simulink model "CubeSatT"  (R2024b)
settings: Solver=ode8  StartTime=0.0  StopTime=10000.0  FixedStep=0.01  RelTol=1e-3
undefined symbols (not defined in the file or in its folder): act, env, flag, IC, orb, sat, sens
libraries: matrix_library x15, simulink_extras x5
(part 2 of 3)

== system CubeSatT/Real World/DKE (Dynamics Kinematics Environment)/Kinematics/Kepler Integrator1 ==
  Add : Sum  Inputs=+-
  Add1 : Sum
  Add2 : Sum
  Clock : Clock
  Constant : Constant  Value=IC.theta
  Constant1 : Constant  Value=3/2
  Constant2 : Constant
  Constant3 : Constant  Value=2
  Constant4 : Constant  Value=orb.e
  Constant5 : Constant  Value=2
  Constant6 : Constant
  Constant7 : Constant  Value=IC.OM
  Constant8 : Constant  Value=2*pi
  Cosh : Trigonometry  Operator=cos
  Divide : Product  Inputs=*/
  Gain : Gain  Gain=orb.n
  Gain1 : Gain  Gain=orb.e
  Gain2 : Gain  Gain=orb.OMprec
  Integrator : Integrator  InitialConditionSource=external  WrapState=on  WrappedStateUpperValue=2*pi  WrappedStateLowerValue=0
  Mod : Math  Operator=mod
  Power : Math  Operator=pow
  Power1 : Math  Operator=pow
  Power2 : Math  Operator=pow
  th : Outport
  OM : Outport  Port=2
  wires:
  Constant/1 -> Integrator/2
  Integrator/1 -> Cosh/1, th/1
  Divide/1 -> Integrator/1
  Power/1 -> Divide/2
  Constant1/1 -> Power/2
  Constant2/1 -> Add/1
  Add/1 -> Power/1
  Power1/1 -> Add/2
  Constant3/1 -> Power1/2
  Constant4/1 -> Power1/1
  Gain/1 -> Divide/1
  Power2/1 -> Gain/1
  Constant5/1 -> Power2/2
  Add1/1 -> Power2/1
  Constant6/1 -> Add1/1
  Gain1/1 -> Add1/2
  Cosh/1 -> Gain1/1
  Constant7/1 -> Add2/2
  Gain2/1 -> Add2/1
  Clock/1 -> Gain2/1
  Add2/1 -> Mod/1
  Constant8/1 -> Mod/2
  Mod/1 -> OM/1

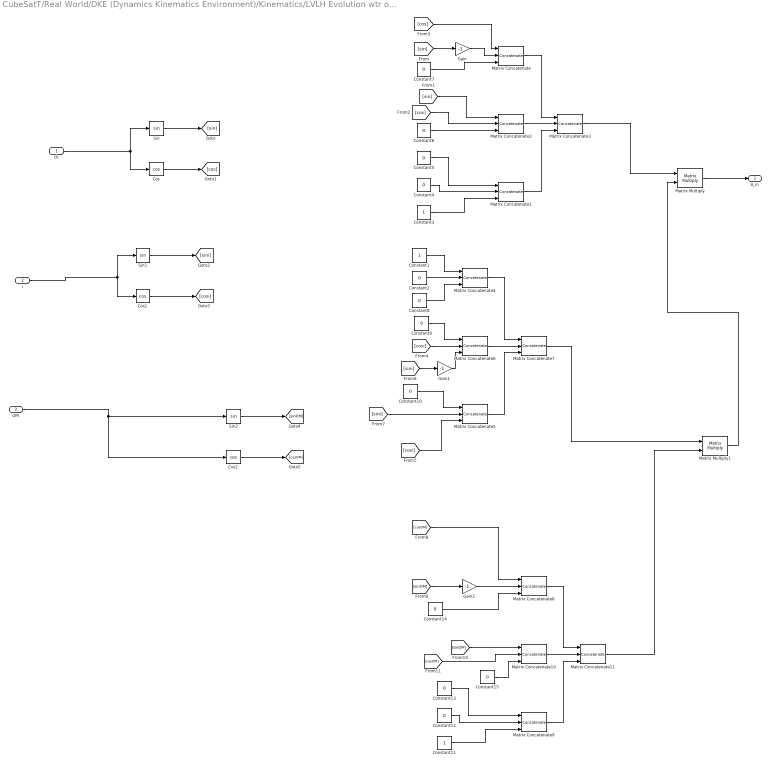
== system CubeSatT/Real World/DKE (Dynamics Kinematics Environment)/Kinematics/LVLH Evolution wtr of Earth ==
  th : Inport
  i : Inport  Port=2
  OM : Inport  Port=3
  Constant1 : Constant
  Constant{2,4..10,12..15} (12 alike) : Constant  Value=0
  Constant11 : Constant
  Constant3 : Constant
  Cos : Trigonometry  Operator=cos
  Cos1 : Trigonometry  Operator=cos
  Cos2 : Trigonometry  Operator=cos
  Gain : Gain  Gain=-1
  Gain1 : Gain  Gain=-1
  Gain2 : Gain  Gain=-1
  Matrix Concatenate{,1..2,4..6,8..10} (9 alike) : Concatenate  NumInputs=3  Mode=Multidimensional array
  Matrix Concatenate11 : Concatenate  NumInputs=3  Mode=Multidimensional array  ConcatenateDimension=2
  Matrix Concatenate3 : Concatenate  NumInputs=3  Mode=Multidimensional array  ConcatenateDimension=2
  Matrix Concatenate7 : Concatenate  NumInputs=3  Mode=Multidimensional array  ConcatenateDimension=2
  Matrix Multiply : Product  Multiplication=Matrix(*)
  Matrix Multiply1 : Product  Multiplication=Matrix(*)
  Sin : Trigonometry
  Sin1 : Trigonometry
  Sin2 : Trigonometry
  A_ln : Outport
  wires:
  Cos/1 -> [cos]
  Matrix Concatenate1/1 -> Matrix Concatenate3/3
  th/1 -> Cos/1, Sin/1
  Matrix Concatenate/1 -> Matrix Concatenate3/1
  Constant5/1 -> Matrix Concatenate1/1
  Constant3/1 -> Matrix Concatenate1/3
  [cos] -> Matrix Concatenate/1
  Sin/1 -> [sin]
  Constant6/1 -> Matrix Concatenate2/3
  Constant7/1 -> Matrix Concatenate/3
  Constant4/1 -> Matrix Concatenate1/2
  Matrix Concatenate2/1 -> Matrix Concatenate3/2
  [cos] -> Matrix Concatenate2/2
  [sin] -> Matrix Concatenate2/1
  Gain/1 -> Matrix Concatenate/2
  [sin] -> Gain/1
  Cos1/1 -> [cosi]
  Sin1/1 -> [sini]
  i/1 -> Cos1/1, Sin1/1
  Matrix Multiply/1 -> A_ln/1
  Matrix Concatenate3/1 -> Matrix Multiply/1
  Matrix Concatenate6/1 -> Matrix Concatenate7/2
  Matrix Concatenate5/1 -> Matrix Concatenate7/3
  Matrix Concatenate4/1 -> Matrix Concatenate7/1
  Constant1/1 -> Matrix Concatenate4/1
  Constant2/1 -> Matrix Concatenate4/2
  Constant8/1 -> Matrix Concatenate4/3
  Constant9/1 -> Matrix Concatenate6/1
  Constant10/1 -> Matrix Concatenate5/1
  [cosi] -> Matrix Concatenate5/3
  [cosi] -> Matrix Concatenate6/2
  [sini] -> Matrix Concatenate5/2
  [sini] -> Gain1/1
  Gain1/1 -> Matrix Concatenate6/3
  Matrix Multiply1/1 -> Matrix Multiply/2
  Matrix Concatenate7/1 -> Matrix Multiply1/1
  OM/1 -> Cos2/1, Sin2/1
  Cos2/1 -> [cosOM]
  Sin2/1 -> [sinOM]
  Matrix Concatenate10/1 -> Matrix Concatenate11/2
  Matrix Concatenate9/1 -> Matrix Concatenate11/3
  Matrix Concatenate8/1 -> Matrix Concatenate11/1
  Matrix Concatenate11/1 -> Matrix Multiply1/2
  Constant13/1 -> Matrix Concatenate9/1
  Constant11/1 -> Matrix Concatenate9/3
  Constant12/1 -> Matrix Concatenate9/2
  Gain2/1 -> Matrix Concatenate8/2
  Constant14/1 -> Matrix Concatenate8/3
  [cosOM] -> Matrix Concatenate8/1
  [sinOM] -> Gain2/1
  [sinOM] -> Matrix Concatenate10/1
  [cosOM] -> Matrix Concatenate10/2
  Constant15/1 -> Matrix Concatenate10/3

== system CubeSatT/Real World/DKE (Dynamics Kinematics Environment)/Kinematics/SpaceCraft position wrt ECI ==
  th : Inport
  OM : Inport  Port=2
  Add : Sum
  Add1 : Sum  Inputs=+-
  Constant{1,7..10,12..15} (9 alike) : Constant  Value=0
  Constant{2..3,11,16} (4 alike) : Constant
  Constant4 : Constant  Value=2
  Constant5 : Constant  Value=orb.e
  Constant6 : Constant  Value=orb.i
  Cos{1..4} (4 alike) : Trigonometry  Operator=cos
  Divide : Product  Inputs=*/
  Gain : Gain  Gain=orb.e
  Gain1 : Gain  Gain=orb.a
  Gain2 : Gain  Gain=-1
  Gain3 : Gain  Gain=-1
  Matrix Concatenate{,4..6,8..10} (7 alike) : Concatenate  NumInputs=3  Mode=Multidimensional array
  Matrix Concatenate11 : Concatenate  NumInputs=3  Mode=Multidimensional array  ConcatenateDimension=2
  Matrix Concatenate7 : Concatenate  NumInputs=3  Mode=Multidimensional array  ConcatenateDimension=2
  Matrix Multiply : Product  Multiplication=Matrix(*)
  Matrix Multiply1 : Product  Multiplication=Matrix(*)
  Power : Math  Operator=pow
  Product2 : Product
  Sin1 : Trigonometry
  Sin2 : Trigonometry
  Sin3 : Trigonometry
  Transpose : Math  Operator=transpose
  r_n : Outport
  wires:
  Cos1/1 -> Matrix Concatenate/1
  th/1 -> Cos2/1, Sin1/1, Cos1/1
  Sin1/1 -> Matrix Concatenate/2
  Product2/1 -> r_n/1
  Divide/1 -> Product2/2
  Constant2/1 -> Add/1
  Add/1 -> Divide/2
  Cos2/1 -> Gain/1
  Gain/1 -> Add/2
  Constant3/1 -> Add1/1
  Power/1 -> Add1/2
  Constant4/1 -> Power/2
  Constant5/1 -> Power/1
  Add1/1 -> Gain1/1
  Gain1/1 -> Divide/1
  Constant6/1 -> Cos3/1, Sin2/1
  Cos3/1 -> [cosi]
  OM/1 -> Cos4/1, Sin3/1
  Sin2/1 -> [sini]
  Sin3/1 -> [sinOM]
  Cos4/1 -> [cosOM]
  Constant1/1 -> Matrix Concatenate/3
  Matrix Multiply/1 -> Product2/1
  Matrix Concatenate/1 -> Matrix Multiply/2
  Transpose/1 -> Matrix Multiply/1
  Constant15/1 -> Matrix Concatenate10/3
  [sinOM] -> Matrix Concatenate10/1
  [sinOM] -> Gain3/1
  Constant13/1 -> Matrix Concatenate9/1
  Gain2/1 -> Matrix Concatenate6/3
  Matrix Concatenate6/1 -> Matrix Concatenate7/2
  Constant14/1 -> Matrix Concatenate8/3
  [sini] -> Gain2/1
  Constant8/1 -> Matrix Concatenate4/3
  Matrix Concatenate4/1 -> Matrix Concatenate7/1
  [cosi] -> Matrix Concatenate5/3
  Constant9/1 -> Matrix Concatenate6/1
  Constant7/1 -> Matrix Concatenate4/2
  Constant10/1 -> Matrix Concatenate5/1
  Matrix Concatenate8/1 -> Matrix Concatenate11/1
  Matrix Concatenate9/1 -> Matrix Concatenate11/3
  Matrix Concatenate7/1 -> Matrix Multiply1/1
  Constant12/1 -> Matrix Concatenate9/2
  [cosi] -> Matrix Concatenate6/2
  Constant11/1 -> Matrix Concatenate9/3
  Constant16/1 -> Matrix Concatenate4/1
  [cosOM] -> Matrix Concatenate10/2
  Gain3/1 -> Matrix Concatenate8/2
  Matrix Concatenate5/1 -> Matrix Concatenate7/3
  [cosOM] -> Matrix Concatenate8/1
  Matrix Concatenate10/1 -> Matrix Concatenate11/2
  [sini] -> Matrix Concatenate5/2
  Matrix Concatenate11/1 -> Matrix Multiply1/2
  Matrix Multiply1/1 -> Transpose/1

== system CubeSatT/Real World/Hardware Models/Actuators/CMG + Control Logic ==
  Mc_b : Inport
  w_mesured : Inport  Port=2
  w : Inport  Port=3
  A assembler : Subsystem
  Add : Sum
  B assembler : Subsystem
  CMG : Subsystem
  Constant3 : Constant  Value=40
  Cross Product : matrix_library/Cross Product
  Degrees to Radians : simulink_extras/Transformations/Degrees to Radians
  Gain : Gain  Gain=-1
  MATLAB Function : MATLAB Function  TreatAsAtomicUnit=on
  Matrix Multiply : Product  Multiplication=Matrix(*)
  hr : Constant  Value=act.cmg.h  VectorParams1D=off
  Mc : Outport
  wires:
  B assembler/1(B) -> MATLAB Function/1(A)
  Mc_b/1 -> Add/1
  CMG/2(Mc) -> Mc/1
  w_mesured/1 -> Cross Product/1
  w/1 -> CMG/2(w)
  Degrees to Radians/1 -> B assembler/1(beta), A assembler/2(beta)
  CMG/1(delta) -> A assembler/1(delta), B assembler/2(delta)
  Matrix Multiply/1 -> Cross Product/2
  Cross Product/1 -> Add/2
  A assembler/1(A) -> Matrix Multiply/1
  hr/1 -> Matrix Multiply/2
  Add/1 -> MATLAB Function/2(B)
  MATLAB Function/1(y) -> Gain/1
  Constant3/1 -> Degrees to Radians/1
  Gain/1 -> CMG/1(delta_dot)

== system CubeSatT/Real World/Hardware Models/Sensors/MAGNETOMETER ==
  note: Missing errors:
      | -SCALE FACTORS ERROR, we can add it to have a more refined model
  B_b : Inport
  Add : Sum
  Constant : Constant  Value=flag.realsensors
  Constant1 : Constant  Value=sens.mag.A_nonorth
  Constant3 : Constant  Value=sens.mag.A_mis
  Demux1 : Demux  Outputs=3
  Matrix Multiply : Product  Multiplication=Matrix(*)
  MatrixMultiply : Product  Multiplication=Matrix(*)
  Mux1 : Mux  Inputs=3
  Noise x : Subsystem
  Noise y : Subsystem
  Noise z : Subsystem
  Switch : Switch  Criteria=u2 > Threshold  SaturateOnIntegerOverflow=off  InputSameDT=off
  "discretization " : ZeroOrderHold  SampleTime=sens.mag.Ts
  quantization : Quantizer  QuantizationInterval=sens.mag.Quant
  saruration : Saturate  UpperLimit=sens.mag.sat(1,1)  LowerLimit=sens.mag.sat(1,2)
  B_meas_b : Outport
  wires:
  Add/1 -> quantization/1
  saruration/1 -> "discretization "/1
  quantization/1 -> saruration/1
  Constant3/1 -> Matrix Multiply/1
  Matrix Multiply/1 -> MatrixMultiply/2
  Constant1/1 -> MatrixMultiply/1
  MatrixMultiply/1 -> Add/1
  Switch/1 -> B_meas_b/1
  Demux1/3 -> Noise z/1(Bz_real)
  B_b/1 -> Demux1/1, Matrix Multiply/2, [B]
  Demux1/1 -> Noise x/1(Bx_real)
  Noise x/1(Out1) -> Mux1/1
  Noise z/1(Out1) -> Mux1/3
  Noise y/1(Out1) -> Mux1/2
  Mux1/1 -> Add/2
  Demux1/2 -> Noise y/1(By_real)
  [B] -> Switch/3
  Constant/1 -> Switch/2
  "discretization "/1 -> Switch/1

== system CubeSatT/Real World/Hardware Models/Sensors/SS Selector ==
  note: Sensor Switch
  note: Validation and Verification Bus Generator
  note: Take care of selecting which Sun Sensor is
      | seeing the sun at a given moment, prioritising the
      | Fine Sensor on the Top panel
      |
      | TODO :
      | Add a variable to switch weights in Wahba's Problem formulation if Fine Sensor is used
      |
      | Change Log
      | Created 21/12/2024
  Fine SS : Inport
  Course SS 1 : Inport  Port=2
  Course SS 2 : Inport  Port=3
  Course SS 3 : Inport  Port=4
  Course SS 4 : Inport  Port=5
  Bus Creator : BusCreator  Inputs=5
  Norm1 : Subsystem
  Norm2 : Subsystem
  Norm3 : Subsystem
  Norm4 : Subsystem
  Switch{,1..3} (4 alike) : Switch  Criteria=u2 ~= 0  SaturateOnIntegerOverflow=off  InputSameDT=off
  Terminator : Terminator
  S_meas_b : Outport
  vv_SS_bus : Outport  Port=2
  wires:
  Fine SS/1 -> [Fine], Norm1/1(Vector)
  Course SS 1/1 -> [Co1], Norm2/1(Vector)
  Course SS 2/1 -> [Co2], Norm3/1(Vector)
  Course SS 3/1 -> [Co3], Norm4/1(Vector)
  Switch/1 -> S_meas_b/1
  Switch1/1 -> Switch/3
  Norm1/1(Norm) -> [FineN]  "norm_r"
  Norm2/1(Norm) -> [Co1N]  "norm_r"
  Norm3/1(Norm) -> [Co2N]  "norm_r"
  Norm4/1(Norm) -> [Co3N]  "norm_r"
  Course SS 4/1 -> Terminator/1, [Co4]  "norm_r"
  Switch2/1 -> Switch1/3
  Switch3/1 -> Switch2/3
  [Co4] -> Switch3/3
  [Fine] -> Switch/1
  [FineN] -> Switch/2
  [Co1] -> Switch1/1
  [Co1N] -> Switch1/2
  [Co2] -> Switch2/1
  [Co2N] -> Switch2/2
  [Co3] -> Switch3/1
  [Co3N] -> Switch3/2
  Bus Creator/1 -> vv_SS_bus/1
  [Fine] -> Bus Creator/1  "Fine_SS"
  [Co1] -> Bus Creator/2  "Co1_SS"
  [Co2] -> Bus Creator/3  "Co2_SS"
  [Co3] -> Bus Creator/4  "Co3_SS"
  [Co4] -> Bus Creator/5  "Co4_SS"

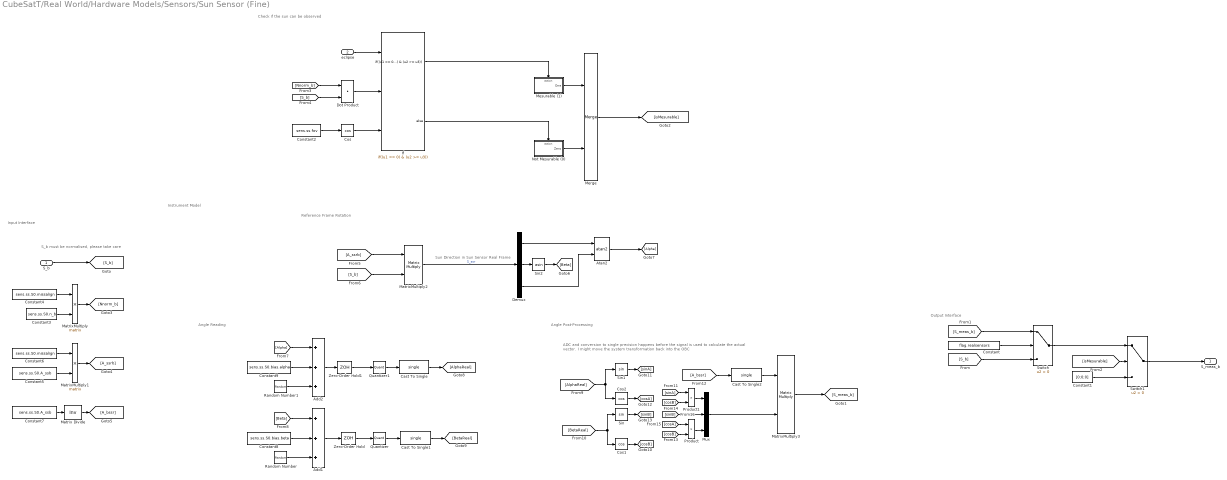
== system CubeSatT/Real World/Hardware Models/Sensors/Sun Sensor (Fine) ==
  note: Instrument Model
  note: Angle Reading
  note: Reference Frame Rotation
  note: ADC and conversion to single precision happens before the signal is used to calculate the actual vector. I might move the system transformation back into the OBC
  note: Sun Direction in Sun Sensor Real Frame
  note: S_b must be normalised, please take care
  note: Input Interface
  note: Output Interface
  note: Check if the sun can be observed
  note: Angle Post-Processing
  S_b : Inport
  eclipse : Inport  Port=2
  Add1 : Sum  Inputs=+++
  Add2 : Sum  Inputs=+++
  Atan2 : Trigonometry  Operator=atan2
  Cast To Single : DataTypeConversion  OutDataTypeStr=single  SaturateOnIntegerOverflow=off  RndMeth=Floor
  Cast To Single1 : DataTypeConversion  OutDataTypeStr=single  SaturateOnIntegerOverflow=off  RndMeth=Floor
  Cast To Single2 : DataTypeConversion  OutDataTypeStr=single  SaturateOnIntegerOverflow=off  RndMeth=Floor
  Constant : Constant  Value=flag.realsensors
  Constant1 : Constant  Value=[0;0;0]
  Constant2 : Constant  Value=sens.ss.fov
  Constant3 : Constant  Value=sens.ss.S0.n_b
  Constant4 : Constant  Value=sens.ss.S0.missalign
  Constant5 : Constant  Value=sens.ss.S0.A_ssb
  Constant6 : Constant  Value=sens.ss.S0.missalign
  Constant7 : Constant  Value=sens.ss.S0.A_ssb
  Constant8 : Constant  Value=sens.ss.S0.bias.beta
  Constant9 : Constant  Value=sens.ss.S0.bias.alpha
  Cos : Trigonometry  Operator=cos
  Cos1 : Trigonometry  Operator=cos
  Cos2 : Trigonometry  Operator=cos
  Demux : Demux  Outputs=3
  Dot Product : DotProduct  OutDataTypeStr=Inherit: Inherit via internal rule
  If : If  NumInputs=3  IfExpression=(u1 == 0) & (u2 >= u3)
  Matrix Divide : Product  Inputs=/  Multiplication=Matrix(*)
  MatrixMultiply{,1..3} (4 alike) : Product  Multiplication=Matrix(*)
  Merge : Merge
  Mesurable (1) : Subsystem  TreatAsAtomicUnit=on
  Mux : Mux  Inputs=3
  Not Mesurable (0) : Subsystem  TreatAsAtomicUnit=on
  Product : Product
  Product1 : Product
  Quantizer : Quantizer  QuantizationInterval=sens.ss.ADC.quanta
  Quantizer1 : Quantizer  QuantizationInterval=sens.ss.ADC.quanta
  Random Number : RandomNumber  Variance=(sens.ss.precision/1.4)^2  Seed=sens.ss.S0.seed.beta  SampleTime=sens.ss.freq
  Random Number1 : RandomNumber  Variance=(sens.ss.precision/1.4)^2  Seed=sens.ss.S0.seed.beta  SampleTime=sens.ss.freq
  Sin : Trigonometry
  Sin1 : Trigonometry
  Sin2 : Trigonometry  Operator=asin
  Switch : Switch  Criteria=u2 > Threshold  SaturateOnIntegerOverflow=off  InputSameDT=off
  Switch1 : Switch  Criteria=u2 > Threshold  SaturateOnIntegerOverflow=off  InputSameDT=off
  Zero-Order Hold : ZeroOrderHold  SampleTime=1/sens.ss.freq
  Zero-Order Hold1 : ZeroOrderHold  SampleTime=1/sens.ss.freq
  S_meas_b : Outport
  wires:
  Constant/1 -> Switch/2
  S_b/1 -> [S_b]
  [S_b] -> Switch/3
  [S_meas_b] -> Switch/1
  eclipse/1 -> If/1
  If/1 -> Mesurable (1)/Action
  If/2 -> Not Mesurable (0)/Action
  Not Mesurable (0)/1(Zero) -> Merge/2
  Mesurable (1)/1(One) -> Merge/1
  Cos/1 -> If/3
  Constant2/1 -> Cos/1
  Dot Product/1 -> If/2
  Merge/1 -> [isMesurable]
  [isMesurable] -> Switch1/2
  [Nnorm_b] -> Dot Product/1
  [S_b] -> Dot Product/2
  Constant4/1 -> MatrixMultiply/1
  MatrixMultiply/1 -> [Nnorm_b]
  Constant3/1 -> MatrixMultiply/2
  Constant1/1 -> Switch1/3
  Switch/1 -> Switch1/1
  Constant6/1 -> MatrixMultiply1/1
  Constant5/1 -> MatrixMultiply1/2
  MatrixMultiply1/1 -> [A_ssrb]
  Constant7/1 -> Matrix Divide/1
  Matrix Divide/1 -> [A_bssr]
  [A_ssrb] -> MatrixMultiply2/1
  [S_b] -> MatrixMultiply2/2
  MatrixMultiply2/1 -> Demux/1  "S_ssr"
  Demux/1 -> Atan2/1
  Demux/3 -> Atan2/2
  Sin2/1 -> [Beta]
  Add2/1 -> Zero-Order Hold1/1
  Add1/1 -> Zero-Order Hold/1
  Quantizer1/1 -> Cast To Single/1
  Zero-Order Hold1/1 -> Quantizer1/1
  Quantizer/1 -> Cast To Single1/1
  Zero-Order Hold/1 -> Quantizer/1
  [Alpha] -> Add2/1
  [Beta] -> Add1/1
  Constant8/1 -> Add1/2
  Constant9/1 -> Add2/2
  Cast To Single/1 -> [AlphaReal]
  Cast To Single1/1 -> [BetaReal]
  Random Number/1 -> Add1/3
  Random Number1/1 -> Add2/3
  Switch1/1 -> S_meas_b/1
  MatrixMultiply3/1 -> [S_meas_b]
  Mux/1 -> MatrixMultiply3/2
  Cast To Single2/1 -> MatrixMultiply3/1
  [A_bssr] -> Cast To Single2/1
  [BetaReal] -> Cos1/1, Sin/1
  Atan2/1 -> [Alpha]
  [AlphaReal] -> Cos2/1, Sin1/1
  Product/1 -> Mux/3
  Product1/1 -> Mux/1
  Demux/2 -> Sin2/1
  Sin1/1 -> [sinA]
  Cos2/1 -> [cosA]
  [sinA] -> Product1/1
  Cos1/1 -> [cosB]
  [cosB] -> Product/2
  [cosB] -> Product1/2
  [cosA] -> Product/1
  Sin/1 -> [sinB]
  [sinB] -> Mux/2

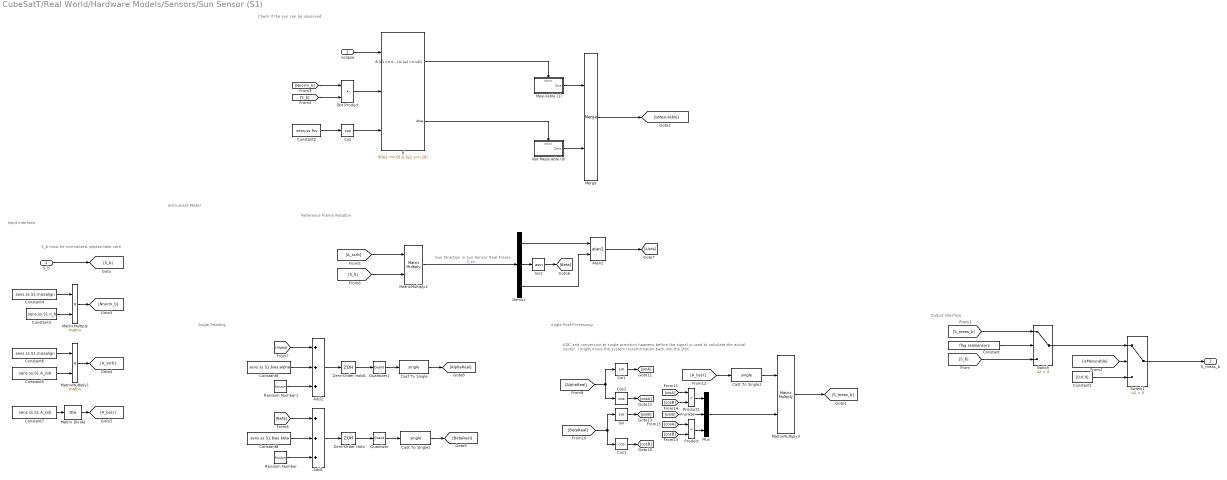
== system CubeSatT/Real World/Hardware Models/Sensors/Sun Sensor (S1) ==
  note: Instrument Model
  note: Angle Reading
  note: Reference Frame Rotation
  note: ADC and conversion to single precision happens before the signal is used to calculate the actual vector. I might move the system transformation back into the OBC
  note: Sun Direction in Sun Sensor Real Frame
  note: S_b must be normalised, please take care
  note: Input Interface
  note: Output Interface
  note: Check if the sun can be observed
  note: Angle Post-Processing
  S_b : Inport
  eclipse : Inport  Port=2
  Add1 : Sum  Inputs=+++
  Add2 : Sum  Inputs=+++
  Atan2 : Trigonometry  Operator=atan2
  Cast To Single : DataTypeConversion  OutDataTypeStr=single  SaturateOnIntegerOverflow=off  RndMeth=Floor
  Cast To Single1 : DataTypeConversion  OutDataTypeStr=single  SaturateOnIntegerOverflow=off  RndMeth=Floor
  Cast To Single2 : DataTypeConversion  OutDataTypeStr=single  SaturateOnIntegerOverflow=off  RndMeth=Floor
  Constant : Constant  Value=flag.realsensors
  Constant1 : Constant  Value=[0;0;0]
  Constant2 : Constant  Value=sens.ss.fov
  Constant3 : Constant  Value=sens.ss.S1.n_b  VectorParams1D=off
  Constant4 : Constant  Value=sens.ss.S1.missalign
  Constant5 : Constant  Value=sens.ss.S1.A_ssb
  Constant6 : Constant  Value=sens.ss.S1.missalign
  Constant7 : Constant  Value=sens.ss.S1.A_ssb
  Constant8 : Constant  Value=sens.ss.S1.bias.beta
  Constant9 : Constant  Value=sens.ss.S1.bias.alpha
  Cos : Trigonometry  Operator=cos
  Cos1 : Trigonometry  Operator=cos
  Cos2 : Trigonometry  Operator=cos
  Demux : Demux  Outputs=3
  Dot Product : DotProduct  OutDataTypeStr=Inherit: Inherit via internal rule
  If : If  NumInputs=3  IfExpression=(u1 == 0) & (u2 >= u3)
  Matrix Divide : Product  Inputs=/  Multiplication=Matrix(*)
  MatrixMultiply{,1..3} (4 alike) : Product  Multiplication=Matrix(*)
  Merge : Merge
  Mesurable (1) : Subsystem  TreatAsAtomicUnit=on
  Mux : Mux  Inputs=3
  Not Mesurable (0) : Subsystem  TreatAsAtomicUnit=on
  Product : Product
  Product1 : Product
  Quantizer : Quantizer  QuantizationInterval=sens.ss.ADC.quanta
  Quantizer1 : Quantizer  QuantizationInterval=sens.ss.ADC.quanta
  Random Number : RandomNumber  Variance=(sens.ss.precision/1.4)^2  Seed=sens.ss.S0.seed.beta  SampleTime=sens.ss.freq
  Random Number1 : RandomNumber  Variance=(sens.ss.precision/1.4)^2  Seed=sens.ss.S0.seed.beta  SampleTime=sens.ss.freq
  Sin : Trigonometry
  Sin1 : Trigonometry
  Sin2 : Trigonometry  Operator=asin
  Switch : Switch  Criteria=u2 > Threshold  SaturateOnIntegerOverflow=off  InputSameDT=off
  Switch1 : Switch  Criteria=u2 > Threshold  SaturateOnIntegerOverflow=off  InputSameDT=off
  Zero-Order Hold : ZeroOrderHold  SampleTime=1/sens.ss.freq
  Zero-Order Hold1 : ZeroOrderHold  SampleTime=1/sens.ss.freq
  S_meas_b : Outport
  wires:
  Constant/1 -> Switch/2
  S_b/1 -> [S_b]
  [S_b] -> Switch/3
  [S_meas_b] -> Switch/1
  eclipse/1 -> If/1
  If/1 -> Mesurable (1)/Action
  If/2 -> Not Mesurable (0)/Action
  Not Mesurable (0)/1(Zero) -> Merge/2
  Mesurable (1)/1(One) -> Merge/1
  Cos/1 -> If/3
  Constant2/1 -> Cos/1
  Dot Product/1 -> If/2
  Merge/1 -> [isMesurable]
  [isMesurable] -> Switch1/2
  [Nnorm_b] -> Dot Product/1
  [S_b] -> Dot Product/2
  Constant4/1 -> MatrixMultiply/1
  MatrixMultiply/1 -> [Nnorm_b]
  Constant3/1 -> MatrixMultiply/2
  Constant1/1 -> Switch1/3
  Switch/1 -> Switch1/1
  Constant6/1 -> MatrixMultiply1/1
  Constant5/1 -> MatrixMultiply1/2
  MatrixMultiply1/1 -> [A_ssrb]
  Constant7/1 -> Matrix Divide/1
  Matrix Divide/1 -> [A_bssr]
  [A_ssrb] -> MatrixMultiply2/1
  [S_b] -> MatrixMultiply2/2
  MatrixMultiply2/1 -> Demux/1  "S_ssr"
  Demux/1 -> Atan2/1
  Demux/3 -> Atan2/2
  Sin2/1 -> [Beta]
  Add2/1 -> Zero-Order Hold1/1
  Add1/1 -> Zero-Order Hold/1
  Quantizer1/1 -> Cast To Single/1
  Zero-Order Hold1/1 -> Quantizer1/1
  Quantizer/1 -> Cast To Single1/1
  Zero-Order Hold/1 -> Quantizer/1
  [Alpha] -> Add2/1
  [Beta] -> Add1/1
  Constant8/1 -> Add1/2
  Constant9/1 -> Add2/2
  Cast To Single/1 -> [AlphaReal]
  Cast To Single1/1 -> [BetaReal]
  Random Number/1 -> Add1/3
  Random Number1/1 -> Add2/3
  Switch1/1 -> S_meas_b/1
  MatrixMultiply3/1 -> [S_meas_b]
  Mux/1 -> MatrixMultiply3/2
  Cast To Single2/1 -> MatrixMultiply3/1
  [A_bssr] -> Cast To Single2/1
  [BetaReal] -> Cos1/1, Sin/1
  Atan2/1 -> [Alpha]
  [AlphaReal] -> Cos2/1, Sin1/1
  Product/1 -> Mux/3
  Product1/1 -> Mux/1
  Demux/2 -> Sin2/1
  Sin1/1 -> [sinA]
  Cos2/1 -> [cosA]
  [sinA] -> Product1/1
  Cos1/1 -> [cosB]
  [cosB] -> Product/2
  [cosB] -> Product1/2
  [cosA] -> Product/1
  Sin/1 -> [sinB]
  [sinB] -> Mux/2

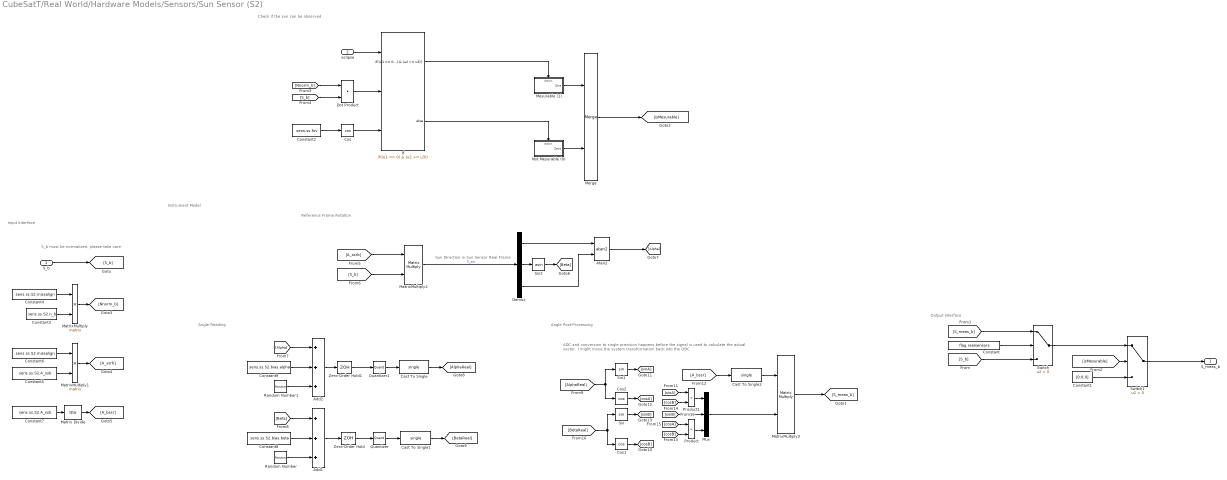
== system CubeSatT/Real World/Hardware Models/Sensors/Sun Sensor (S2) ==
  note: Instrument Model
  note: Angle Reading
  note: Reference Frame Rotation
  note: ADC and conversion to single precision happens before the signal is used to calculate the actual vector. I might move the system transformation back into the OBC
  note: Sun Direction in Sun Sensor Real Frame
  note: S_b must be normalised, please take care
  note: Input Interface
  note: Output Interface
  note: Check if the sun can be observed
  note: Angle Post-Processing
  S_b : Inport
  eclipse : Inport  Port=2
  Add1 : Sum  Inputs=+++
  Add2 : Sum  Inputs=+++
  Atan2 : Trigonometry  Operator=atan2
  Cast To Single : DataTypeConversion  OutDataTypeStr=single  SaturateOnIntegerOverflow=off  RndMeth=Floor
  Cast To Single1 : DataTypeConversion  OutDataTypeStr=single  SaturateOnIntegerOverflow=off  RndMeth=Floor
  Cast To Single2 : DataTypeConversion  OutDataTypeStr=single  SaturateOnIntegerOverflow=off  RndMeth=Floor
  Constant : Constant  Value=flag.realsensors
  Constant1 : Constant  Value=[0;0;0]
  Constant2 : Constant  Value=sens.ss.fov
  Constant3 : Constant  Value=sens.ss.S2.n_b
  Constant4 : Constant  Value=sens.ss.S2.missalign
  Constant5 : Constant  Value=sens.ss.S2.A_ssb
  Constant6 : Constant  Value=sens.ss.S2.missalign  VectorParams1D=off
  Constant7 : Constant  Value=sens.ss.S2.A_ssb
  Constant8 : Constant  Value=sens.ss.S2.bias.beta
  Constant9 : Constant  Value=sens.ss.S2.bias.alpha
  Cos : Trigonometry  Operator=cos
  Cos1 : Trigonometry  Operator=cos
  Cos2 : Trigonometry  Operator=cos
  Demux : Demux  Outputs=3
  Dot Product : DotProduct  OutDataTypeStr=Inherit: Inherit via internal rule
  If : If  NumInputs=3  IfExpression=(u1 == 0) & (u2 >= u3)
  Matrix Divide : Product  Inputs=/  Multiplication=Matrix(*)
  MatrixMultiply{,1..3} (4 alike) : Product  Multiplication=Matrix(*)
  Merge : Merge
  Mesurable (1) : Subsystem  TreatAsAtomicUnit=on
  Mux : Mux  Inputs=3
  Not Mesurable (0) : Subsystem  TreatAsAtomicUnit=on
  Product : Product
  Product1 : Product
  Quantizer : Quantizer  QuantizationInterval=sens.ss.ADC.quanta
  Quantizer1 : Quantizer  QuantizationInterval=sens.ss.ADC.quanta
  Random Number : RandomNumber  Variance=(sens.ss.precision/1.4)^2  Seed=sens.ss.S0.seed.beta  SampleTime=sens.ss.freq
  Random Number1 : RandomNumber  Variance=(sens.ss.precision/1.4)^2  Seed=sens.ss.S0.seed.beta  SampleTime=sens.ss.freq
  Sin : Trigonometry
  Sin1 : Trigonometry
  Sin2 : Trigonometry  Operator=asin
  Switch : Switch  Criteria=u2 > Threshold  SaturateOnIntegerOverflow=off  InputSameDT=off
  Switch1 : Switch  Criteria=u2 > Threshold  SaturateOnIntegerOverflow=off  InputSameDT=off
  Zero-Order Hold : ZeroOrderHold  SampleTime=1/sens.ss.freq
  Zero-Order Hold1 : ZeroOrderHold  SampleTime=1/sens.ss.freq
  S_meas_b : Outport
  wires:
  Constant/1 -> Switch/2
  S_b/1 -> [S_b]
  [S_b] -> Switch/3
  [S_meas_b] -> Switch/1
  eclipse/1 -> If/1
  If/1 -> Mesurable (1)/Action
  If/2 -> Not Mesurable (0)/Action
  Not Mesurable (0)/1(Zero) -> Merge/2
  Mesurable (1)/1(One) -> Merge/1
  Cos/1 -> If/3
  Constant2/1 -> Cos/1
  Dot Product/1 -> If/2
  Merge/1 -> [isMesurable]
  [isMesurable] -> Switch1/2
  [Nnorm_b] -> Dot Product/1
  [S_b] -> Dot Product/2
  Constant4/1 -> MatrixMultiply/1
  MatrixMultiply/1 -> [Nnorm_b]
  Constant3/1 -> MatrixMultiply/2
  Constant1/1 -> Switch1/3
  Switch/1 -> Switch1/1
  Constant6/1 -> MatrixMultiply1/1
  Constant5/1 -> MatrixMultiply1/2
  MatrixMultiply1/1 -> [A_ssrb]
  Constant7/1 -> Matrix Divide/1
  Matrix Divide/1 -> [A_bssr]
  [A_ssrb] -> MatrixMultiply2/1
  [S_b] -> MatrixMultiply2/2
  MatrixMultiply2/1 -> Demux/1  "S_ssr"
  Demux/1 -> Atan2/1
  Demux/3 -> Atan2/2
  Sin2/1 -> [Beta]
  Add2/1 -> Zero-Order Hold1/1
  Add1/1 -> Zero-Order Hold/1
  Quantizer1/1 -> Cast To Single/1
  Zero-Order Hold1/1 -> Quantizer1/1
  Quantizer/1 -> Cast To Single1/1
  Zero-Order Hold/1 -> Quantizer/1
  [Alpha] -> Add2/1
  [Beta] -> Add1/1
  Constant8/1 -> Add1/2
  Constant9/1 -> Add2/2
  Cast To Single/1 -> [AlphaReal]
  Cast To Single1/1 -> [BetaReal]
  Random Number/1 -> Add1/3
  Random Number1/1 -> Add2/3
  Switch1/1 -> S_meas_b/1
  MatrixMultiply3/1 -> [S_meas_b]
  Mux/1 -> MatrixMultiply3/2
  Cast To Single2/1 -> MatrixMultiply3/1
  [A_bssr] -> Cast To Single2/1
  [BetaReal] -> Cos1/1, Sin/1
  Atan2/1 -> [Alpha]
  [AlphaReal] -> Cos2/1, Sin1/1
  Product/1 -> Mux/3
  Product1/1 -> Mux/1
  Demux/2 -> Sin2/1
  Sin1/1 -> [sinA]
  Cos2/1 -> [cosA]
  [sinA] -> Product1/1
  Cos1/1 -> [cosB]
  [cosB] -> Product/2
  [cosB] -> Product1/2
  [cosA] -> Product/1
  Sin/1 -> [sinB]
  [sinB] -> Mux/2

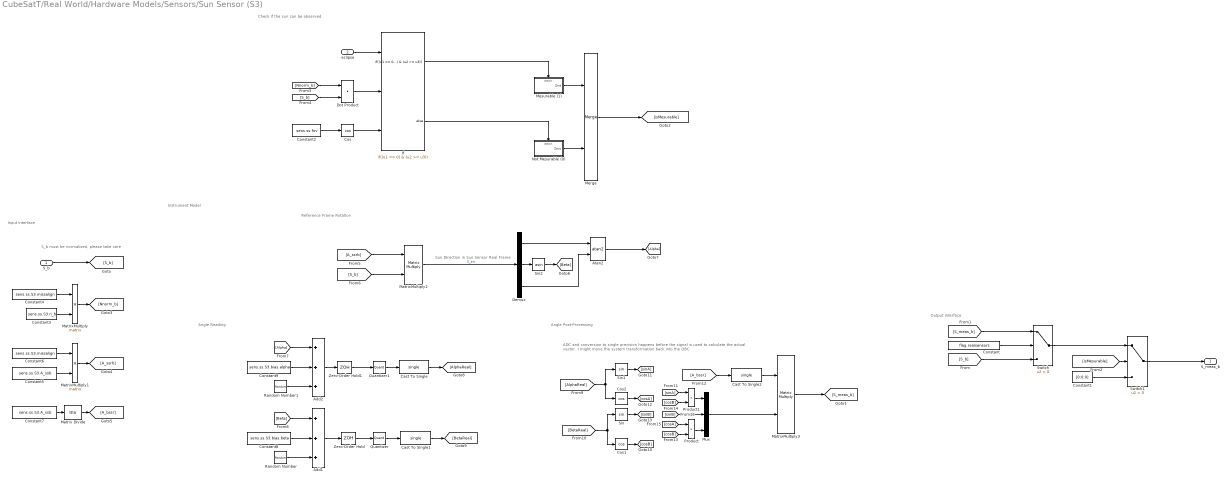
== system CubeSatT/Real World/Hardware Models/Sensors/Sun Sensor (S3) ==
  note: Instrument Model
  note: Angle Reading
  note: Reference Frame Rotation
  note: ADC and conversion to single precision happens before the signal is used to calculate the actual vector. I might move the system transformation back into the OBC
  note: Sun Direction in Sun Sensor Real Frame
  note: S_b must be normalised, please take care
  note: Input Interface
  note: Output Interface
  note: Check if the sun can be observed
  note: Angle Post-Processing
  S_b : Inport
  eclipse : Inport  Port=2
  Add1 : Sum  Inputs=+++
  Add2 : Sum  Inputs=+++
  Atan2 : Trigonometry  Operator=atan2
  Cast To Single : DataTypeConversion  OutDataTypeStr=single  SaturateOnIntegerOverflow=off  RndMeth=Floor
  Cast To Single1 : DataTypeConversion  OutDataTypeStr=single  SaturateOnIntegerOverflow=off  RndMeth=Floor
  Cast To Single2 : DataTypeConversion  OutDataTypeStr=single  SaturateOnIntegerOverflow=off  RndMeth=Floor
  Constant : Constant  Value=flag.realsensors
  Constant1 : Constant  Value=[0;0;0]
  Constant2 : Constant  Value=sens.ss.fov
  Constant3 : Constant  Value=sens.ss.S3.n_b
  Constant4 : Constant  Value=sens.ss.S3.missalign
  Constant5 : Constant  Value=sens.ss.S3.A_ssb
  Constant6 : Constant  Value=sens.ss.S3.missalign
  Constant7 : Constant  Value=sens.ss.S3.A_ssb
  Constant8 : Constant  Value=sens.ss.S3.bias.beta
  Constant9 : Constant  Value=sens.ss.S3.bias.alpha
  Cos : Trigonometry  Operator=cos
  Cos1 : Trigonometry  Operator=cos
  Cos2 : Trigonometry  Operator=cos
  Demux : Demux  Outputs=3
  Dot Product : DotProduct  OutDataTypeStr=Inherit: Inherit via internal rule
  If : If  NumInputs=3  IfExpression=(u1 == 0) & (u2 >= u3)
  Matrix Divide : Product  Inputs=/  Multiplication=Matrix(*)
  MatrixMultiply{,1..3} (4 alike) : Product  Multiplication=Matrix(*)
  Merge : Merge
  Mesurable (1) : Subsystem  TreatAsAtomicUnit=on
  Mux : Mux  Inputs=3
  Not Mesurable (0) : Subsystem  TreatAsAtomicUnit=on
  Product : Product
  Product1 : Product
  Quantizer : Quantizer  QuantizationInterval=sens.ss.ADC.quanta
  Quantizer1 : Quantizer  QuantizationInterval=sens.ss.ADC.quanta
  Random Number : RandomNumber  Variance=(sens.ss.precision/1.4)^2  Seed=sens.ss.S0.seed.beta  SampleTime=sens.ss.freq
  Random Number1 : RandomNumber  Variance=(sens.ss.precision/1.4)^2  Seed=sens.ss.S0.seed.beta  SampleTime=sens.ss.freq
  Sin : Trigonometry
  Sin1 : Trigonometry
  Sin2 : Trigonometry  Operator=asin
  Switch : Switch  Criteria=u2 > Threshold  SaturateOnIntegerOverflow=off  InputSameDT=off
  Switch1 : Switch  Criteria=u2 > Threshold  SaturateOnIntegerOverflow=off  InputSameDT=off
  Zero-Order Hold : ZeroOrderHold  SampleTime=1/sens.ss.freq
  Zero-Order Hold1 : ZeroOrderHold  SampleTime=1/sens.ss.freq
  S_meas_b : Outport
  wires:
  Constant/1 -> Switch/2
  S_b/1 -> [S_b]
  [S_b] -> Switch/3
  [S_meas_b] -> Switch/1
  eclipse/1 -> If/1
  If/1 -> Mesurable (1)/Action
  If/2 -> Not Mesurable (0)/Action
  Not Mesurable (0)/1(Zero) -> Merge/2
  Mesurable (1)/1(One) -> Merge/1
  Cos/1 -> If/3
  Constant2/1 -> Cos/1
  Dot Product/1 -> If/2
  Merge/1 -> [isMesurable]
  [isMesurable] -> Switch1/2
  [Nnorm_b] -> Dot Product/1
  [S_b] -> Dot Product/2
  Constant4/1 -> MatrixMultiply/1
  MatrixMultiply/1 -> [Nnorm_b]
  Constant3/1 -> MatrixMultiply/2
  Constant1/1 -> Switch1/3
  Switch/1 -> Switch1/1
  Constant6/1 -> MatrixMultiply1/1
  Constant5/1 -> MatrixMultiply1/2
  MatrixMultiply1/1 -> [A_ssrb]
  Constant7/1 -> Matrix Divide/1
  Matrix Divide/1 -> [A_bssr]
  [A_ssrb] -> MatrixMultiply2/1
  [S_b] -> MatrixMultiply2/2
  MatrixMultiply2/1 -> Demux/1  "S_ssr"
  Demux/1 -> Atan2/1
  Demux/3 -> Atan2/2
  Sin2/1 -> [Beta]
  Add2/1 -> Zero-Order Hold1/1
  Add1/1 -> Zero-Order Hold/1
  Quantizer1/1 -> Cast To Single/1
  Zero-Order Hold1/1 -> Quantizer1/1
  Quantizer/1 -> Cast To Single1/1
  Zero-Order Hold/1 -> Quantizer/1
  [Alpha] -> Add2/1
  [Beta] -> Add1/1
  Constant8/1 -> Add1/2
  Constant9/1 -> Add2/2
  Cast To Single/1 -> [AlphaReal]
  Cast To Single1/1 -> [BetaReal]
  Random Number/1 -> Add1/3
  Random Number1/1 -> Add2/3
  Switch1/1 -> S_meas_b/1
  MatrixMultiply3/1 -> [S_meas_b]
  Mux/1 -> MatrixMultiply3/2
  Cast To Single2/1 -> MatrixMultiply3/1
  [A_bssr] -> Cast To Single2/1
  [BetaReal] -> Cos1/1, Sin/1
  Atan2/1 -> [Alpha]
  [AlphaReal] -> Cos2/1, Sin1/1
  Product/1 -> Mux/3
  Product1/1 -> Mux/1
  Demux/2 -> Sin2/1
  Sin1/1 -> [sinA]
  Cos2/1 -> [cosA]
  [sinA] -> Product1/1
  Cos1/1 -> [cosB]
  [cosB] -> Product/2
  [cosB] -> Product1/2
  [cosA] -> Product/1
  Sin/1 -> [sinB]
  [sinB] -> Mux/2

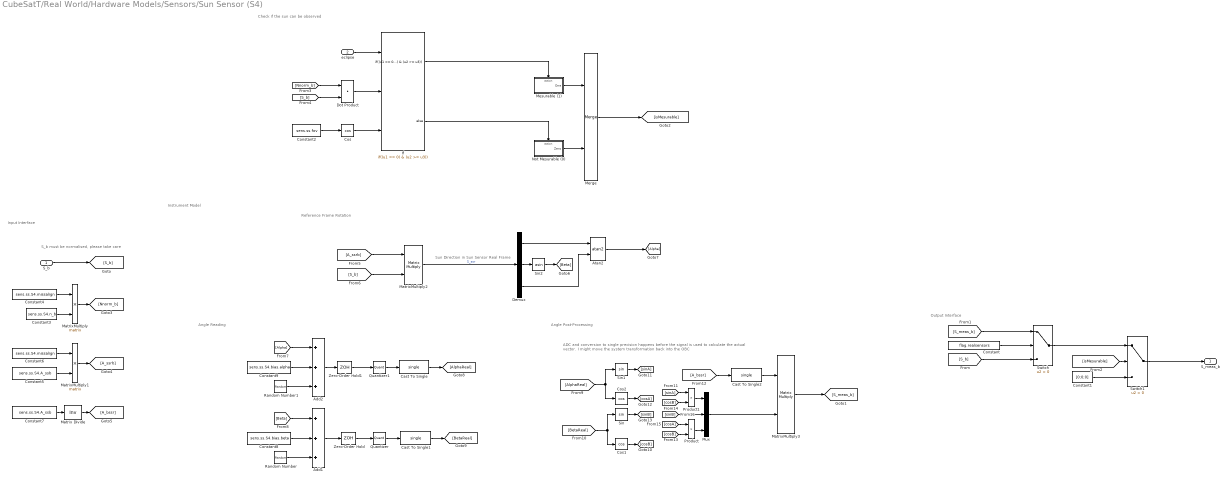
== system CubeSatT/Real World/Hardware Models/Sensors/Sun Sensor (S4) ==
  note: Instrument Model
  note: Angle Reading
  note: Reference Frame Rotation
  note: ADC and conversion to single precision happens before the signal is used to calculate the actual vector. I might move the system transformation back into the OBC
  note: Sun Direction in Sun Sensor Real Frame
  note: S_b must be normalised, please take care
  note: Input Interface
  note: Output Interface
  note: Check if the sun can be observed
  note: Angle Post-Processing
  S_b : Inport
  eclipse : Inport  Port=2
  Add1 : Sum  Inputs=+++
  Add2 : Sum  Inputs=+++
  Atan2 : Trigonometry  Operator=atan2
  Cast To Single : DataTypeConversion  OutDataTypeStr=single  SaturateOnIntegerOverflow=off  RndMeth=Floor
  Cast To Single1 : DataTypeConversion  OutDataTypeStr=single  SaturateOnIntegerOverflow=off  RndMeth=Floor
  Cast To Single2 : DataTypeConversion  OutDataTypeStr=single  SaturateOnIntegerOverflow=off  RndMeth=Floor
  Constant : Constant  Value=flag.realsensors
  Constant1 : Constant  Value=[0;0;0]
  Constant2 : Constant  Value=sens.ss.fov
  Constant3 : Constant  Value=sens.ss.S4.n_b
  Constant4 : Constant  Value=sens.ss.S4.missalign
  Constant5 : Constant  Value=sens.ss.S4.A_ssb
  Constant6 : Constant  Value=sens.ss.S4.missalign
  Constant7 : Constant  Value=sens.ss.S4.A_ssb
  Constant8 : Constant  Value=sens.ss.S4.bias.beta
  Constant9 : Constant  Value=sens.ss.S4.bias.alpha
  Cos : Trigonometry  Operator=cos
  Cos1 : Trigonometry  Operator=cos
  Cos2 : Trigonometry  Operator=cos
  Demux : Demux  Outputs=3
  Dot Product : DotProduct  OutDataTypeStr=Inherit: Inherit via internal rule
  If : If  NumInputs=3  IfExpression=(u1 == 0) & (u2 >= u3)
  Matrix Divide : Product  Inputs=/  Multiplication=Matrix(*)
  MatrixMultiply{,1..3} (4 alike) : Product  Multiplication=Matrix(*)
  Merge : Merge
  Mesurable (1) : Subsystem  TreatAsAtomicUnit=on
  Mux : Mux  Inputs=3
  Not Mesurable (0) : Subsystem  TreatAsAtomicUnit=on
  Product : Product
  Product1 : Product
  Quantizer : Quantizer  QuantizationInterval=sens.ss.ADC.quanta
  Quantizer1 : Quantizer  QuantizationInterval=sens.ss.ADC.quanta
  Random Number : RandomNumber  Variance=(sens.ss.precision/1.4)^2  Seed=sens.ss.S0.seed.beta  SampleTime=sens.ss.freq
  Random Number1 : RandomNumber  Variance=(sens.ss.precision/1.4)^2  Seed=sens.ss.S0.seed.beta  SampleTime=sens.ss.freq
  Sin : Trigonometry
  Sin1 : Trigonometry
  Sin2 : Trigonometry  Operator=asin
  Switch : Switch  Criteria=u2 > Threshold  SaturateOnIntegerOverflow=off  InputSameDT=off
  Switch1 : Switch  Criteria=u2 > Threshold  SaturateOnIntegerOverflow=off  InputSameDT=off
  Zero-Order Hold : ZeroOrderHold  SampleTime=1/sens.ss.freq
  Zero-Order Hold1 : ZeroOrderHold  SampleTime=1/sens.ss.freq
  S_meas_b : Outport
  wires:
  Constant/1 -> Switch/2
  S_b/1 -> [S_b]
  [S_b] -> Switch/3
  [S_meas_b] -> Switch/1
  eclipse/1 -> If/1
  If/1 -> Mesurable (1)/Action
  If/2 -> Not Mesurable (0)/Action
  Not Mesurable (0)/1(Zero) -> Merge/2
  Mesurable (1)/1(One) -> Merge/1
  Cos/1 -> If/3
  Constant2/1 -> Cos/1
  Dot Product/1 -> If/2
  Merge/1 -> [isMesurable]
  [isMesurable] -> Switch1/2
  [Nnorm_b] -> Dot Product/1
  [S_b] -> Dot Product/2
  Constant4/1 -> MatrixMultiply/1
  MatrixMultiply/1 -> [Nnorm_b]
  Constant3/1 -> MatrixMultiply/2
  Constant1/1 -> Switch1/3
  Switch/1 -> Switch1/1
  Constant6/1 -> MatrixMultiply1/1
  Constant5/1 -> MatrixMultiply1/2
  MatrixMultiply1/1 -> [A_ssrb]
  Constant7/1 -> Matrix Divide/1
  Matrix Divide/1 -> [A_bssr]
  [A_ssrb] -> MatrixMultiply2/1
  [S_b] -> MatrixMultiply2/2
  MatrixMultiply2/1 -> Demux/1  "S_ssr"
  Demux/1 -> Atan2/1
  Demux/3 -> Atan2/2
  Sin2/1 -> [Beta]
  Add2/1 -> Zero-Order Hold1/1
  Add1/1 -> Zero-Order Hold/1
  Quantizer1/1 -> Cast To Single/1
  Zero-Order Hold1/1 -> Quantizer1/1
  Quantizer/1 -> Cast To Single1/1
  Zero-Order Hold/1 -> Quantizer/1
  [Alpha] -> Add2/1
  [Beta] -> Add1/1
  Constant8/1 -> Add1/2
  Constant9/1 -> Add2/2
  Cast To Single/1 -> [AlphaReal]
  Cast To Single1/1 -> [BetaReal]
  Random Number/1 -> Add1/3
  Random Number1/1 -> Add2/3
  Switch1/1 -> S_meas_b/1
  MatrixMultiply3/1 -> [S_meas_b]
  Mux/1 -> MatrixMultiply3/2
  Cast To Single2/1 -> MatrixMultiply3/1
  [A_bssr] -> Cast To Single2/1
  [BetaReal] -> Cos1/1, Sin/1
  Atan2/1 -> [Alpha]
  [AlphaReal] -> Cos2/1, Sin1/1
  Product/1 -> Mux/3
  Product1/1 -> Mux/1
  Demux/2 -> Sin2/1
  Sin1/1 -> [sinA]
  Cos2/1 -> [cosA]
  [sinA] -> Product1/1
  Cos1/1 -> [cosB]
  [cosB] -> Product/2
  [cosB] -> Product1/2
  [cosA] -> Product/1
  Sin/1 -> [sinB]
  [sinB] -> Mux/2

== system CubeSatT/OBC/Guidance/Sun Pointing Guidance/Attitude Error/[q (-)] ==
  q* : Inport
  Matrix Concatenate : Concatenate  Mode=Multidimensional array  ConcatenateDimension=2
  Xi(q) : Subsystem
  Out2 : Outport
  wires:
  Matrix Concatenate/1 -> Out2/1
  q*/1 -> Xi(q)/1(In1), Matrix Concatenate/2
  Xi(q)/1(Out1) -> Matrix Concatenate/1

== system CubeSatT/OBC/Guidance/Sun Pointing Guidance/Attitude Error/q* ==
  note: Evaluate the quaternion coniugate
  q : Inport
  Demux : Demux
  Gain : Gain  Gain=-1
  Gain1 : Gain  Gain=-1
  Gain2 : Gain  Gain=-1
  Mux : Mux
  q* : Outport
  wires:
  Mux/1 -> q*/1
  Demux/4 -> Mux/4
  q/1 -> Demux/1
  Demux/1 -> Gain/1
  Demux/2 -> Gain1/1
  Demux/3 -> Gain2/1
  Gain/1 -> Mux/1
  Gain1/1 -> Mux/2
  Gain2/1 -> Mux/3

== system CubeSatT/OBC/Navigation/Subsystem1/K matrix computing/Trace ==
  In1 : Inport
  Extract Diagonal : matrix_library/Extract Diagonal
  Sum of Elements : Sum  Inputs=+
  Out1 : Outport
  wires:
  In1/1 -> Extract Diagonal/1
  Extract Diagonal/1 -> Sum of Elements/1
  Sum of Elements/1 -> Out1/1

== system CubeSatT/OBC/Reference/Sun Direction Circular Orbit/Normaliser (with Built In safety)/Norm1 ==
  Vector : Inport
  Add : Sum  Inputs=+++
  Demux : Demux  Outputs=3
  Sqrt : Sqrt
  Square : Math  Operator=square
  Square1 : Math  Operator=square
  Square2 : Math  Operator=square
  Norm : Outport
  wires:
  Square/1 -> Add/1
  Add/1 -> Sqrt/1
  Demux/3 -> Square1/1
  Square2/1 -> Add/2
  Square1/1 -> Add/3
  Demux/1 -> Square/1
  Demux/2 -> Square2/1
  Vector/1 -> Demux/1
  Sqrt/1 -> Norm/1

== system CubeSatT/OBC/Reference/Sun Direction Circular Orbit/Normaliser (with Built In safety)/Protected Division ==
  Vector : Inport
  Norm : Inport  Port=2
  Constant : Constant  Value=eps
  Divide : Product  Inputs=*/
  Switch : Switch  Criteria=u2 ~= 0  SaturateOnIntegerOverflow=off  InputSameDT=off
  Out1 : Outport
  wires:
  Divide/1 -> Out1/1
  Vector/1 -> Divide/1
  Norm/1 -> Switch/1, Switch/2
  Switch/1 -> Divide/2
  Constant/1 -> Switch/3

== system CubeSatT/Real World/DKE (Dynamics Kinematics Environment)/Environment/Conical Shadow Model/Eclipse (1) ==
  Action Port : ActionPort  ActionPortLabel=if(u1 < u2)
  Constant : Constant
  One : Outport
  wires:
  Constant/1 -> One/1

== system CubeSatT/Real World/DKE (Dynamics Kinematics Environment)/Environment/Conical Shadow Model/Norm ==
  Vector : Inport
  Add : Sum  Inputs=+++
  Demux : Demux  Outputs=3
  Sqrt : Sqrt
  Square : Math  Operator=square
  Square1 : Math  Operator=square
  Square2 : Math  Operator=square
  Norm : Outport
  wires:
  Square/1 -> Add/1
  Add/1 -> Sqrt/1
  Demux/3 -> Square1/1
  Square2/1 -> Add/2
  Square1/1 -> Add/3
  Demux/1 -> Square/1
  Demux/2 -> Square2/1
  Vector/1 -> Demux/1
  Sqrt/1 -> Norm/1

== system CubeSatT/Real World/DKE (Dynamics Kinematics Environment)/Environment/Conical Shadow Model/NotEclipse (0) ==
  Action Port : ActionPort  ActionPortLabel=else
  Constant : Constant  Value=0
  Zero : Outport
  wires:
  Constant/1 -> Zero/1

== system CubeSatT/Real World/DKE (Dynamics Kinematics Environment)/Environment/Magnetic Field order 1/Norm ==
  Vector : Inport
  Add : Sum  Inputs=+++
  Demux : Demux  Outputs=3
  Sqrt : Sqrt
  Square : Math  Operator=square
  Square1 : Math  Operator=square
  Square2 : Math  Operator=square
  Norm : Outport
  wires:
  Square/1 -> Add/1
  Add/1 -> Sqrt/1
  Demux/3 -> Square1/1
  Square2/1 -> Add/2
  Square1/1 -> Add/3
  Demux/1 -> Square/1
  Demux/2 -> Square2/1
  Vector/1 -> Demux/1
  Sqrt/1 -> Norm/1

== system CubeSatT/Real World/DKE (Dynamics Kinematics Environment)/Environment/Magnetic Field order 1/Norm1 ==
  Vector : Inport
  Add : Sum  Inputs=+++
  Demux : Demux  Outputs=3
  Sqrt : Sqrt
  Square : Math  Operator=square
  Square1 : Math  Operator=square
  Square2 : Math  Operator=square
  Norm : Outport
  wires:
  Square/1 -> Add/1
  Add/1 -> Sqrt/1
  Demux/3 -> Square1/1
  Square2/1 -> Add/2
  Square1/1 -> Add/3
  Demux/1 -> Square/1
  Demux/2 -> Square2/1
  Vector/1 -> Demux/1
  Sqrt/1 -> Norm/1

== system CubeSatT/Real World/DKE (Dynamics Kinematics Environment)/Environment/Magnetic Field order 1/Norm2 ==
  Vector : Inport
  Add : Sum  Inputs=+++
  Demux : Demux  Outputs=3
  Sqrt : Sqrt
  Square : Math  Operator=square
  Square1 : Math  Operator=square
  Square2 : Math  Operator=square
  Norm : Outport
  wires:
  Square/1 -> Add/1
  Add/1 -> Sqrt/1
  Demux/3 -> Square1/1
  Square2/1 -> Add/2
  Square1/1 -> Add/3
  Demux/1 -> Square/1
  Demux/2 -> Square2/1
  Vector/1 -> Demux/1
  Sqrt/1 -> Norm/1

== system CubeSatT/Real World/DKE (Dynamics Kinematics Environment)/Environment/Perturbations/Gravity Gradient Torque ==
  A_bl : Inport
  r_n : Inport  Port=2
  Constant : Constant  Value=[0; 0; 0]
  Constant1 : Constant  Value=flag.gg
  Constant3 : Constant  Value=3
  Constant5 : Constant  Value=env.Earth.mass
  Constant6 : Constant  Value=env.G
  Constant7 : Constant  Value=[1; 0; 0]
  Constant8 : Constant  Value=sat.I
  Cross Product1 : matrix_library/Cross Product
  Divide1 : Product  Inputs=**/
  Gain : Gain  Gain=3
  Norm : Subsystem
  Power : Math  Operator=pow
  Product1 : Product
  Product2 : Product  Multiplication=Matrix(*)
  Product3 : Product  Multiplication=Matrix(*)
  Switch : Switch  Criteria=u2 > Threshold  SaturateOnIntegerOverflow=off  InputSameDT=off
  T_gg : Outport
  wires:
  A_bl/1 -> Product2/1
  Product3/1 -> Cross Product1/2
  Product2/1 -> [c]
  Constant8/1 -> Product3/1
  Product1/1 -> Cross Product1/1
  [c] -> Product1/1
  [c] -> Product3/2
  Constant6/1 -> Divide1/1
  Constant5/1 -> Divide1/2
  r_n/1 -> Norm/1(Vector)
  Constant7/1 -> Product2/2
  Constant3/1 -> Power/2
  Power/1 -> Divide1/3
  Divide1/1 -> Gain/1
  Gain/1 -> Product1/2
  Constant/1 -> Switch/3
  Switch/1 -> T_gg/1
  Cross Product1/1 -> Switch/1
  Constant1/1 -> Switch/2
  Norm/1(Norm) -> Power/1  "norm_r"

== system CubeSatT/Real World/DKE (Dynamics Kinematics Environment)/Environment/Perturbations/Magnetic Field Torque ==
  r_n : Inport
  A(B/N) : Inport  Port=2
  Clock : Clock
  Constant : Constant  Value=env.mag.dgrf2020
  Constant1 : Constant  Value=env.Earth.R
  Constant2 : Constant  Value=3
  Constant3 : Constant  Value=env.Earth.magInclination
  Constant4 : Constant  Value=3
  Constant5 : Constant  Value=flag.mag
  Constant6 : Constant  Value=[0; 0; 0]
  Constant7 : Constant  Value=sat.jB
  Cos : Trigonometry  Operator=cos
  Cos1 : Trigonometry  Operator=cos
  Cross Product : matrix_library/Cross Product
  Divide : Product  Inputs=***/
  Divide1 : Product  Inputs=*/
  Divide2 : Product  Inputs=*/
  Dot Product : DotProduct  OutDataTypeStr=Inherit: Inherit via internal rule
  Gain : Gain  Gain=3
  Gain1 : Gain  Gain=env.Earth.omega
  Mux : Mux  Inputs=3
  Norm : Subsystem
  Norm1 : Subsystem
  Norm2 : Subsystem
  Power : Math  Operator=pow
  Power1 : Math  Operator=pow
  Product : Product
  Product1 : Product
  Product2 : Product
  Product9 : Product  Multiplication=Matrix(*)
  Sin : Trigonometry
  Sin1 : Trigonometry
  Sqrt : Sqrt
  Square : Math  Operator=square
  Subtract : Sum  Inputs=+-
  Sum of Elements : Sum  Inputs=+
  Switch : Switch  Criteria=u2 > Threshold  SaturateOnIntegerOverflow=off  InputSameDT=off
  T_mag : Outport
  wires:
  Constant/1 -> Square/1
  Square/1 -> Sum of Elements/1
  Sum of Elements/1 -> Sqrt/1
  Constant1/1 -> Power/1
  Constant2/1 -> Power/2
  Sqrt/1 -> Divide/2
  Power/1 -> Divide/3
  Constant4/1 -> Power1/2
  Power1/1 -> Divide/4
  Norm/1(Norm) -> Power1/1  "norm_r"
  r_n/1 -> Norm2/1(Vector), Divide2/1, [rr]
  [rr] -> Norm/1(Vector)
  [rr_hat] -> Dot Product/2
  Subtract/1 -> Divide/1
  [mm] -> Subtract/2
  Dot Product/1 -> Product/2
  Product/1 -> Gain/1
  Gain/1 -> Subtract/1
  [rr_hat] -> Product/1
  [mm] -> Dot Product/1
  Mux/1 -> Norm1/1(Vector), Divide1/1
  Cos/1 -> Mux/3
  Constant3/1 -> Sin/1, Cos/1
  Clock/1 -> Gain1/1
  Sin/1 -> Product2/2, Product1/2
  Product1/1 -> Mux/2
  Product2/1 -> Mux/1
  Cos1/1 -> Product2/1
  Gain1/1 -> Cos1/1, Sin1/1
  Sin1/1 -> Product1/1
  Divide/1 -> Product9/2
  Norm1/1(Norm) -> Divide1/2  "norm_r"
  Divide1/1 -> [mm]
  Norm2/1(Norm) -> Divide2/2  "norm_r"
  Divide2/1 -> [rr_hat]
  Constant5/1 -> Switch/2
  Constant6/1 -> Switch/3
  Cross Product/1 -> Switch/1
  A(B/N)/1 -> Product9/1
  Constant7/1 -> Cross Product/1
  Switch/1 -> T_mag/1
  Product9/1 -> Cross Product/2

== system CubeSatT/Real World/DKE (Dynamics Kinematics Environment)/Environment/Perturbations/Solar Radiation Pressure Torque ==
  S_b : Inport
  Constant : Constant  Value=flag.srp
  Constant1 : Constant  Value=[0; 0; 0]
  Constant3 : Constant  Value=ones(6,1)-sat.rho_s
  Constant4 : Constant  Value=sat.rho_s
  Constant5 : Constant  Value=sat.rho_d
  Gain1 : Gain  Gain=-env.dis.P
  Gain2 : Gain  Gain=2
  Gain3 : Gain  Gain=2/3
  Matrix Concatenate : Concatenate  NumInputs=3  Mode=Multidimensional array
  Matrix Concatenate2 : Concatenate  NumInputs=3  Mode=Multidimensional array
  MatrixMultiply : Product  Multiplication=Matrix(*)
  Normaliser : Subsystem
  Product{,1,3..4} (4 alike) : Product
  Product2 : Product  Multiplication=Matrix(*)
  Reshape : Reshape
  Saturation : Saturate  UpperLimit=1  LowerLimit=0
  Sum1 : Sum  Inputs=+|+
  Sum2 : Sum  Inputs=+|+
  Switch : Switch  Criteria=u2 > Threshold  SaturateOnIntegerOverflow=off  InputSameDT=off
  Transpose : Math  Operator=transpose
  Transpose2 : Math  Operator=transpose
  Transpose3 : Math  Operator=transpose
  cross product r x F : Subsystem
  surface : Constant  Value=sat.A
  unit vector matrix : Constant  Value=sat.n_b
  T_srp : Outport
  wires:
  Product3/1 -> Transpose3/1
  Saturation/1 -> Product4/2, Product1/1
  Gain3/1 -> Sum1/2
  surface/1 -> Gain1/1
  unit vector matrix/1 -> MatrixMultiply/2, Product/2
  Constant4/1 -> Gain2/1
  Constant3/1 -> Product2/1
  Sum2/1 -> Product3/2
  [S_b] -> Product2/2
  Constant5/1 -> Gain3/1
  Product4/1 -> Sum1/1
  MatrixMultiply/1 -> Saturation/1
  Gain2/1 -> Product4/1
  Product2/1 -> Transpose/1
  S_b/1 -> Normaliser/1(Vector)
  Normaliser/1(Out1) -> Transpose2/1
  Transpose2/1 -> MatrixMultiply/1, [S_b]
  Product/1 -> Sum2/2
  Transpose/1 -> Sum2/1
  Transpose3/1 -> cross product r x F/1(F_srp)
  Gain1/1 -> Product1/2
  Sum1/1 -> Matrix Concatenate/3, Matrix Concatenate/1, Matrix Concatenate/2
  Matrix Concatenate/1 -> Product/1
  Product1/1 -> Matrix Concatenate2/3, Matrix Concatenate2/2, Matrix Concatenate2/1
  Matrix Concatenate2/1 -> Product3/1
  cross product r x F/1(Out1) -> Switch/1
  Constant/1 -> Switch/2
  Switch/1 -> Reshape/1
  Constant1/1 -> Switch/3
  Reshape/1 -> T_srp/1

== system CubeSatT/Real World/DKE (Dynamics Kinematics Environment)/Environment/Sun Direction Circular Orbit/Normaliser (with Built In safety) ==
  Vector : Inport
  Constant : Constant  Value=[0; 0; 0]  VectorParams1D=off
  Norm1 : Subsystem
  Protected Division : Subsystem
  Switch : Switch  Criteria=u2 ~= 0  SaturateOnIntegerOverflow=off  InputSameDT=off
  Out1 : Outport
  wires:
  Norm1/1(Norm) -> Switch/2, Protected Division/2(Norm)  "norm_r"
  Switch/1 -> Out1/1
  Protected Division/1(Out1) -> Switch/1
  Vector/1 -> Protected Division/1(Vector), Norm1/1(Vector)
  Constant/1 -> Switch/3

== system CubeSatT/Real World/DKE (Dynamics Kinematics Environment)/Kinematics/EulerKinematicsdelay/312 Propagator ==
  IC : Inport
  w_b : Inport  Port=2
  Reset : Inport  Port=3
  Cos1 : Trigonometry  Operator=cos
  Cos2 : Trigonometry  Operator=cos
  Demux : Demux  Outputs=3
  Demux1 : Demux  Outputs=3
  Divide1 : Product  Inputs=*/
  Integrator1 : Integrator  ExternalReset=either  InitialConditionSource=external  WrapState=on  WrappedStateUpperValue=2*pi  WrappedStateLowerValue=0  ShowStatePort=on
  Integrator2 : Integrator  ExternalReset=either  InitialConditionSource=external  WrapState=on  ShowStatePort=on
  Integrator3 : Integrator  ExternalReset=either  InitialConditionSource=external  WrapState=on  WrappedStateUpperValue=2*pi  WrappedStateLowerValue=0  ShowStatePort=on
  Mux : Mux  Inputs=3
  Mux1 : Mux  Inputs=3
  Product{1..7} (7 alike) : Product
  Sin : Trigonometry
  Subtract : Sum  Inputs=+-
  Subtract1 : Sum
  Subtract2 : Sum  Inputs=+-
  Subtract3 : Sum  Inputs=+-
  Tan : Trigonometry  Operator=tan
  EA : Outport
  Out1 : Outport  Port=2
  wires:
  Product6/1 -> Subtract3/2
  Product5/1 -> Subtract3/1
  Product4/1 -> Subtract1/2
  Integrator3/1 -> [theta3]
  [wz] -> Product5/1
  Mux/1 -> EA/1
  Product7/1 -> Subtract2/2
  Cos1/1 -> [cosPsi]
  [theta3] -> Sin/1, Cos1/1
  [cosPsi] -> Product1/2
  Demux/2 -> [wy]
  Tan/1 -> [tanThe]
  Product2/1 -> Subtract/2
  [wz] -> Product3/1
  [tanThe] -> Product7/2
  Cos2/1 -> [cosThe]
  [cosPsi] -> Product5/2
  Divide1/1 -> Integrator1/1
  Subtract1/1 -> Integrator2/1
  Demux/3 -> [wz]
  [theta1] -> Mux/1
  Subtract/1 -> Divide1/1
  Demux/1 -> [wx]
  Subtract2/1 -> Integrator3/1
  [theta2] -> Tan/1, Cos2/1
  [wy] -> Subtract2/1
  Integrator1/1 -> [theta1]
  Integrator2/1 -> [theta2]
  [wx] -> Product4/1
  [sinPsi] -> Product2/2
  w_b/1 -> Demux/1
  Subtract3/1 -> Product7/1
  Product3/1 -> Subtract1/1
  [theta2] -> Mux/2
  [sinPsi] -> Product3/2
  [theta3] -> Mux/3
  [sinPsi] -> Product6/2
  [wx] -> Product6/1
  [wx] -> Product2/1
  [cosPsi] -> Product4/2
  [wz] -> Product1/1
  Product1/1 -> Subtract/1
  [cosThe] -> Divide1/2
  Sin/1 -> [sinPsi]
  Demux1/1 -> Integrator1/3
  Demux1/2 -> Integrator2/3
  Demux1/3 -> Integrator3/3
  IC/1 -> Demux1/1
  Reset/1 -> Integrator2/2, Integrator3/2, Integrator1/2
  Integrator3/State -> Mux1/3
  Integrator2/State -> Mux1/2
  Integrator1/State -> Mux1/1
  Mux1/1 -> Out1/1
